simulink model "FCE_TX_RX"  (R2015a)
settings: Solver=ode45  StartTime=0.0  StopTime=2  RelTol=1e-3
libraries: dsparch4 x1
settings Model: Creator=dhairya  LastModifiedBy=dhairya

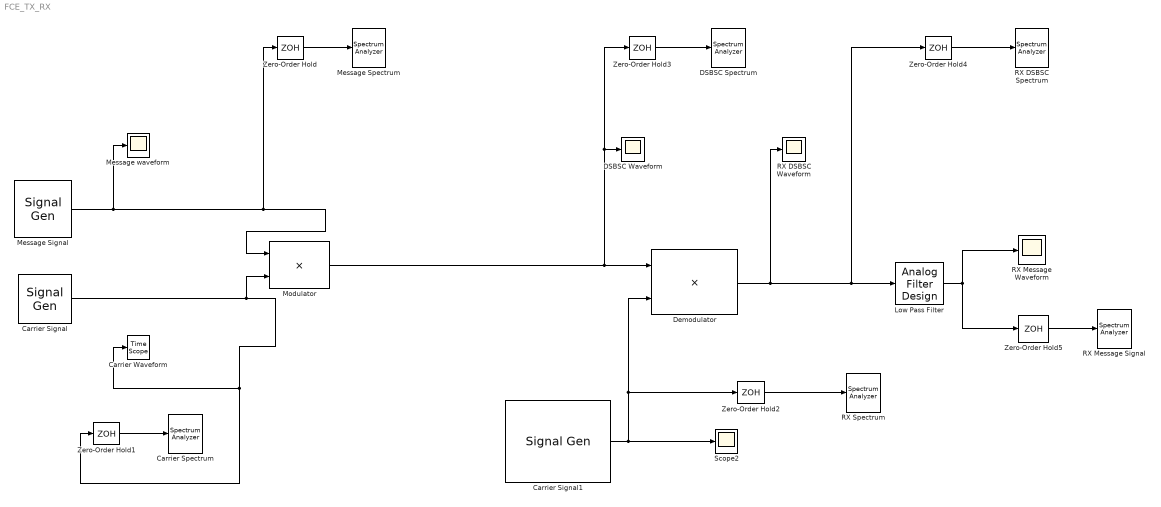
== system FCE_TX_RX ==
  Carrier Waveform : TimeScope
  Carrier Signal : SignalGenerator  Frequency=1500
  Carrier Signal1 : SignalGenerator  Frequency=1500
  Carrier Spectrum : SpectrumAnalyzer
  DSBSC Waveform : Scope
      settings: TimeRange=0.05  YMin=-2  YMax=2  SaveName=ScopeData3
  DSBSC Spectrum : SpectrumAnalyzer
  Demodulator : Product
  Low Pass Filter : dsparch4/Analog Filter Design  method=Butterworth  filttype=Lowpass  N=8  Wlo=2*pi*400  Whi=80  Rp=2  Rs=40
  Message waveform : Scope
      settings: TickLabels=on  TimeRange=0.05  YMin=-2  YMax=2  ScrollMode=on
  Message Signal : SignalGenerator  Frequency=200
  Message Spectrum : SpectrumAnalyzer
  Modulator : Product
  RX DSBSC Waveform : Scope
      settings: TimeRange=0.05  YMin=-2  YMax=2  SaveName=ScopeData4
  RX DSBSC Spectrum : SpectrumAnalyzer
  RX Message Waveform : Scope
      settings: TimeRange=0.05  YMin=-0.5  YMax=0.5  SaveName=ScopeData5
  RX Message Signal : SpectrumAnalyzer
  RX Spectrum : SpectrumAnalyzer
  Scope2 : Scope
      settings: SaveName=ScopeData2
  Zero-Order Hold : ZeroOrderHold  SampleTime=1/4000
  Zero-Order Hold{1..5} (5 alike) : ZeroOrderHold  SampleTime=1/30000
  wires:
  Zero-Order Hold/1 -> Message Spectrum/1
  Message Signal/1 -> Modulator/1, Zero-Order Hold/1, Message waveform/1
  Zero-Order Hold1/1 -> Carrier Spectrum/1
  Carrier Signal/1 -> Zero-Order Hold1/1, Carrier Waveform/1, Modulator/2
  Zero-Order Hold2/1 -> RX Spectrum/1
  Carrier Signal1/1 -> Demodulator/2, Zero-Order Hold2/1, Scope2/1
  Zero-Order Hold3/1 -> DSBSC Spectrum/1
  Modulator/1 -> Zero-Order Hold3/1, DSBSC Waveform/1, Demodulator/1
  Zero-Order Hold4/1 -> RX DSBSC Spectrum/1
  Demodulator/1 -> Zero-Order Hold4/1, Low Pass Filter/1, RX DSBSC Waveform/1
  Zero-Order Hold5/1 -> RX Message Signal/1
  Low Pass Filter/1 -> RX Message Waveform/1, Zero-Order Hold5/1
